simulink model "asservisement_corrige"  (R2019a)
settings: Solver=VariableStepAuto  StartTime=0.0  StopTime=60000000  RelTol=1e-3
model workspace (MAT data in the model file):
  Cx = 0.84
  S = 0.04
libraries: fl_lib x9, nesl_utility x8, sh_lib x5, ee_lib x4, shared3dof x1, simulink x1, dspswit3 x1
settings Model: Creator=Paul  LastModifiedBy=Paul

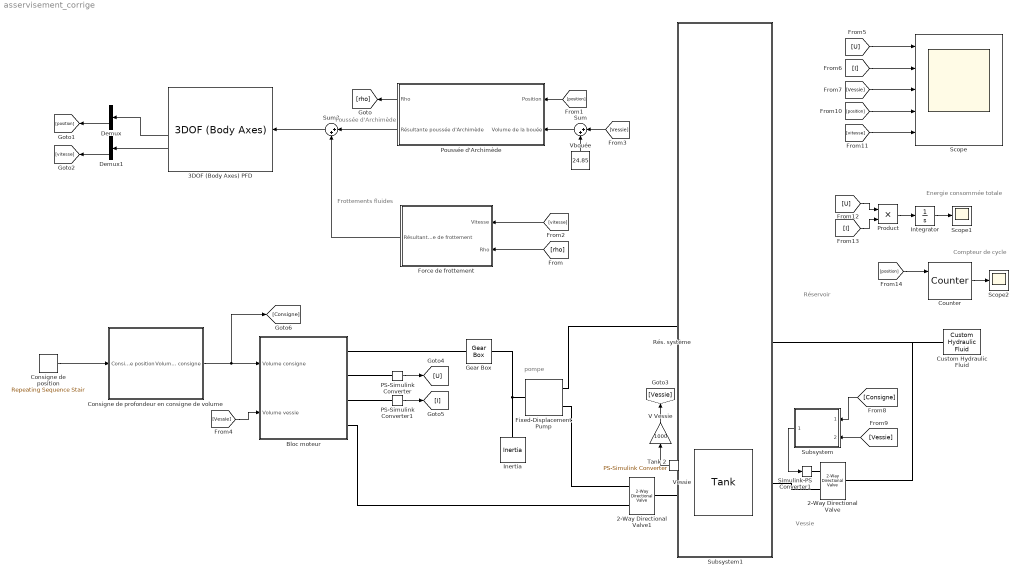
== system asservisement_corrige ==
  note: Vessie
  note: pompe
  note: Energie consommée totale
  note: Compteur de cycle
  note: Poussée d'Archimède
  note: Réservoir
  note: Frottements fluides
  2-Way Directional Valve : sh_lib/Valves/Directional Valves/2-Way Directional Valve  mdl_type=1  area_max=2e-3 m^2  opening_max=0.05 m  opening_tab=[-.002, 0, .002, .005, .015] m  area_tab=[1e-09, 2.0352e-07, 4.0736e-05, .00011438, .00034356] m^2  pressure_tab=[-10000000, -5000000, -2000000, 2000000, 5000000, 10000000] Pa  flow_rate_tab=[-1e-07, -7.0711e-08, -4.4721e-08, 4.4721e-08, 7.0711e-08, 1e-07; -2.0352e-05, -1.4391e-05, -9.1017e-06, 9.1017e-06, 1.4391e-05, 2.0352e-05; -.0040736, -.0028805, -.0018218, .0018218, .0028805, .0040736; -.011438, -.0080879, -.0051152, .0051152, .0080879, .011438; -.034356, -.024293, -.015364, .015364, .024293, .034356] m^3/s  interp_method=1  extrap_method=1  C_d=0.7  x_0=0 m  A_leak=1e-15 m^2  lam_spec=1  B_lam=0.999  Re_cr=12
      settings: SourceProductName=Simscape Fluids  SourceProductBaseCode=SH
  2-Way Directional Valve1 : sh_lib/Valves/Directional Valves/2-Way Directional Valve  mdl_type=1  area_max=2e-2 m^2  opening_max=0.05 m  opening_tab=[-.002, 0, .002, .005, .015] m  area_tab=[1e-09, 2.0352e-07, 4.0736e-05, .00011438, .00034356] m^2  pressure_tab=[-10000000, -5000000, -2000000, 2000000, 5000000, 10000000] Pa  flow_rate_tab=[-1e-07, -7.0711e-08, -4.4721e-08, 4.4721e-08, 7.0711e-08, 1e-07; -2.0352e-05, -1.4391e-05, -9.1017e-06, 9.1017e-06, 1.4391e-05, 2.0352e-05; -.0040736, -.0028805, -.0018218, .0018218, .0028805, .0040736; -.011438, -.0080879, -.0051152, .0051152, .0080879, .011438; -.034356, -.024293, -.015364, .015364, .024293, .034356] m^3/s  interp_method=1  extrap_method=1  C_d=0.7  x_0=0 m  A_leak=1e-15 m^2  lam_spec=1  B_lam=0.999  Re_cr=12
      settings: SourceProductName=Simscape Fluids  SourceProductBaseCode=SH
  "3DOF (Body Axes) PFD " : shared3dof/3DOF (Body Axes)  units=Metric (MKS)  mtype=Fixed  v_ini=0  theta_ini=0  alpha_ini=0  pos_ini=[0 0]  q_ini=0  mass=26  mass_e=0.5  mass_f=3.0  Iyy=1.0  Iyy_e=0.5  Iyy_f=3.0  g_in=Internal  g=9.81  vre_flag=on  abi_flag=off  aMode=0  vel_statename=''  theta_statename=''  pos_statename=''  q_statename=''  mass_statename=''
      settings: SourceProductName=Aerospace Blockset  SourceProductBaseCode=AE
  "Bloc moteur " : Subsystem
  "Consigne de position " : simulink/Sources/Repeating Sequence Stair  OutValues=[0 1000 1000 1000 4000 0].'  tsamp=100000  OutMin=[]  OutMax=[]  OutDataTypeStr=double  OutputDataTypeScalingMode=double  OutDataType=fixdt(0,8)  ConRadixGroup=Best Precision: Vector-wise  OutScaling=2^-12
  Consigne de profondeur en consigne de volume : Subsystem
  Counter : dspswit3/Counter  Direction=Up  CountEvent=Falling edge  CounterSize=User defined  MaxCount=255  InitialCount=0  Output=Count  HitValue=32  ResetInput=on  SamplesPerFrame=1  Ts=1  CntDtype=double  HitDtype=Logical
  Custom Hydraulic Fluid : fl_lib/Hydraulic/Hydraulic Utilities/Custom Hydraulic Fluid  density=850 kg/m^3  viscosity_kin=18e-6 m^2/s  bulk=0.8e9 Pa  alpha=0.005  range_error=2
      settings: SourceProductName=Simscape  SourceProductBaseCode=SS
  Demux : Demux  Outputs=2
  Demux1 : Demux  Outputs=2
  Fixed-Displacement Pump : sh_lib/Pumps and Motors/Fixed-Displacement Pump  D=15 cm^3/rev  loss_spec=1  w_nominal=4 rpm  pr_nominal=400e5 Pa  visc_nominal=18 cSt  dens_nominal=900 kg/m^3  efficiency_vol=0.92  no_load_torque=0.05 N*m  torque_pressure_coeff=0.6e-6 N*m/Pa  p_diff_eff_TLU=[100000, 1000000, 2000000] Pa  omega_eff_TLU=[25, 50, 100, 200, 300, 400] rad/s  vol_eff_TLU=[.816, .908, .954, .977, .981, .984; .325, .663, .831, .916, .925, .946; .137, .568, .78, .892, .893, .91]  mech_eff_TLU=[.996, .996, .996, .996, .996, .996; .988, .989, .989, .989, .989, .99; .981, .981, .982, .982, .983, .984]  p_diff_loss_TLU=[100000, 1000000, 2000000] Pa  omega_loss_TLU=[25, 50, 100, 200, 300, 400] rad/s  vol_loss_TLU=[.023, .023, .023, .023, .0285, .032; .0844, .0842, .0845, .084, .1125, .108; .1079, .108, .11, .108, .1605, .18] * 1e-3 m^3/s  mech_loss_TLU=[.002, .002, .002, .002, .002, .002; .0607, .0556, .0556, .0556, .0556, .0505; .1937, .1937, .1833, .1833, .1729, .1626] N*m  pressure_threshold=1e5 Pa  omega_threshold=10 rad/s  quadrant_check=0  pressure_check=0  min_valid_pressure=0 Pa  vol_eff_min=1e-3  vol_eff_max=1  mech_eff_min=1e-3  mech_eff_max=1
      settings: SourceProductName=Simscape Fluids  SourceProductBaseCode=SH
  Force de frottement : Subsystem
  Gear Box : fl_lib/Mechanical/Mechanisms/Gear Box  ratio=1000  t_in_specify=off  t_in_priority=None  t_in=0 N*m  t_in_nominal_specify=off  t_in_nominal_unit=N*m  t_in_nominal_value=1  t_out_specify=off  t_out_priority=None  t_out=0 N*m  t_out_nominal_specify=off  t_out_nominal_unit=N*m  t_out_nominal_value=1
  Inertia : fl_lib/Mechanical/Rotational Elements/Inertia  inertia=200 g*cm^2  w_specify=off  w_priority=High  w=0 rad/s  w_nominal_specify=off  w_nominal_unit=rad/s  w_nominal_value=1  t_specify=off  t_priority=None  t=0 N*m  t_nominal_specify=off  t_nominal_unit=N*m  t_nominal_value=1
  Integrator : Integrator
  PS-Simulink Converter : nesl_utility/PS-Simulink Converter  PhysicalDomain=network_engine_domain  SubClassName=ps_output  LeftPortType=input  RightPortType=output  PseudoPeriodic=off  Frequencies=[]  Unit=1  AffineConversion=off
  PS-Simulink Converter1 : nesl_utility/PS-Simulink Converter  PhysicalDomain=network_engine_domain  SubClassName=ps_output  LeftPortType=input  RightPortType=output  PseudoPeriodic=off  Frequencies=[]  Unit=1  AffineConversion=off
  Poussée d'Archimède : Subsystem
  Product : Product
  Rés. système : sh_lib/Low-Pressure Blocks/Tank  press=1 bar  level_spec=1  tank_area=0.8 m^2  fluid_volume_tab=[0, .0028, .0065, .0114, .0176, .0252, .0344, .0436, .0512, .0574, .0623, .066, .0688, .0707, .072, .0727] m^3  fluid_level_tab=[0, .02, .04, .06, .08, .1, .12, .14, .16, .18, .2, .22, .24, .26, .28, .3] m  interp_method=1  extrap_method=1  pipe_diam=0.02 m  loss_coeff=1.2  g=9.80665 m/s^2  min_level=1e-3 m  fluid_level_check=0  volume_specify=on  volume_priority=High  volume=0 l  volume_nominal_specify=off  volume_nominal_unit=l  volume_nominal_value=1  level_specify=off  level_priority=None  level=0.025 m  level_nominal_specify=off  level_nominal_unit=m  level_nominal_value=1  pipe_diam_A=0.02 m  loss_coeff_A=1.2  height_B=0.8 m  pipe_diam_B=0.02 m  loss_coeff_B=1.2  height_C=0.8 m  pipe_diam_C=0.02 m  loss_coeff_C=1.2
      settings: SourceProductName=Simscape Fluids  SourceProductBaseCode=SH
  Scope : Scope  NumInputPorts=5
  Scope1 : Scope
  Scope2 : Scope
  Simulink-PS Converter1 : nesl_utility/Simulink-PS Converter  PhysicalDomain=network_engine_domain  SubClassName=ps_input  LeftPortType=input  RightPortType=output  PseudoPeriodic=off  Frequencies=[]  NoiseDistribution=none  NoiseParameters=[]  Unit=m  AffineConversion=off  FilteringAndDerivatives=provide  SimscapeFilterOrder=1  InputFilterTimeConstant=0.001  UdotUserProvided=0
  Subsystem : Subsystem
  Subsystem1 : Subsystem
      mask Display: image('D:\Paul\Documents\TIPE\matlab\Les+flotteurs+Argo2.jpg');
  Sum : Sum  Inputs=|++
  Sum3 : Sum  Inputs=|++
  Tank 2 : nesl_utility/PS-Simulink Converter  PhysicalDomain=network_engine_domain  SubClassName=ps_output  LeftPortType=input  RightPortType=output  PseudoPeriodic=off  Frequencies=[]  Unit=1  AffineConversion=off
  V Vessie : Gain  Gain=1000
  Vbouée : Constant  Value=24.85
  Vessie : sh_lib/Low-Pressure Blocks/Tank  press=400 bar  level_spec=1  tank_area=0.8 m^2  fluid_volume_tab=[0, .0028, .0065, .0114, .0176, .0252, .0344, .0436, .0512, .0574, .0623, .066, .0688, .0707, .072, .0727] m^3  fluid_level_tab=[0, .02, .04, .06, .08, .1, .12, .14, .16, .18, .2, .22, .24, .26, .28, .3] m  interp_method=1  extrap_method=1  pipe_diam=0.02 m  loss_coeff=1.2  g=9.80665 m/s^2  min_level=1e-3 m  fluid_level_check=1  volume_specify=on  volume_priority=High  volume=0.45 l  volume_nominal_specify=off  volume_nominal_unit=l  volume_nominal_value=1  level_specify=off  level_priority=None  level=0.025 m  level_nominal_specify=off  level_nominal_unit=m  level_nominal_value=1  pipe_diam_A=0.02 m  loss_coeff_A=1.2  height_B=0.8 m  pipe_diam_B=0.02 m  loss_coeff_B=1.2  height_C=0.8 m  pipe_diam_C=0.02 m  loss_coeff_C=1.2
      settings: SourceProductName=Simscape Fluids  SourceProductBaseCode=SH
  wires:
  [U] -> Product/1
  Tank 2/1 -> V Vessie/1
  [position] -> Scope/4
  Sum/1 -> Poussée d'Archimède/2(Volume de la bouée)
  Demux/2 -> [position]
  Integrator/1 -> Scope1/1
  Vbouée/1 -> Sum/2
  Force de frottement/1(Résultante force de frottement) -> Sum3/2
  Product/1 -> Integrator/1
  PS-Simulink Converter/1 -> [U]
  [Vessie] -> Subsystem/2(Volume vessie)
  Subsystem/1(Consigne vanne) -> Simulink-PS Converter1/1
  "Consigne de position "/1 -> Consigne de profondeur en consigne de volume/1(Consigne de position)
  [rho] -> Force de frottement/2(Rho)
  "3DOF (Body Axes) PFD "/5 -> Demux1/1
  [I] -> Scope/2
  [I] -> Product/2
  Poussée d'Archimède/2(Résultante poussée d'Archimède) -> Sum3/1
  [position] -> Poussée d'Archimède/1(Position)
  V Vessie/1 -> [Vessie]
  Consigne de profondeur en consigne de volume/1(Volume consigne) -> [Consigne], "Bloc moteur "/1(Volume consigne)
  Poussée d'Archimède/1("Rho ") -> [rho]
  Sum3/1 -> "3DOF (Body Axes) PFD "/2
  [U] -> Scope/1
  [Vessie] -> Sum/1
  [Vessie] -> Scope/3
  "3DOF (Body Axes) PFD "/4 -> Demux/1
  [Vessie] -> "Bloc moteur "/2(Volume vessie)
  [vitesse] -> Scope/5
  [vitesse] -> Force de frottement/1(Vitesse)
  PS-Simulink Converter1/1 -> [I]
  [Consigne] -> Subsystem/1(Volume consigne)
  Demux1/2 -> [vitesse]
  [position] -> Counter/1
  Counter/1 -> Scope2/1
  connections:
  Inertia/LConn1 -- Gear Box/RConn1 -- Fixed-Displacement Pump/LConn1
  Rés. système/LConn1 -- 2-Way Directional Valve/RConn1 -- Custom Hydraulic Fluid/RConn1
  2-Way Directional Valve1/LConn2 -- Fixed-Displacement Pump/RConn1
  Rés. système/RConn2 -- Fixed-Displacement Pump/RConn2
  Simulink-PS Converter1/RConn1 -- 2-Way Directional Valve/LConn1
  Vessie/RConn1 -- Tank 2/LConn1
  Vessie/RConn2 -- 2-Way Directional Valve1/RConn1
  "Bloc moteur "/RConn1 -- Gear Box/LConn1
  Vessie/LConn1 -- 2-Way Directional Valve/LConn2
  2-Way Directional Valve1/LConn1 -- "Bloc moteur "/RConn4
  "Bloc moteur "/RConn2 -- PS-Simulink Converter/LConn1
  PS-Simulink Converter1/LConn1 -- "Bloc moteur "/RConn3

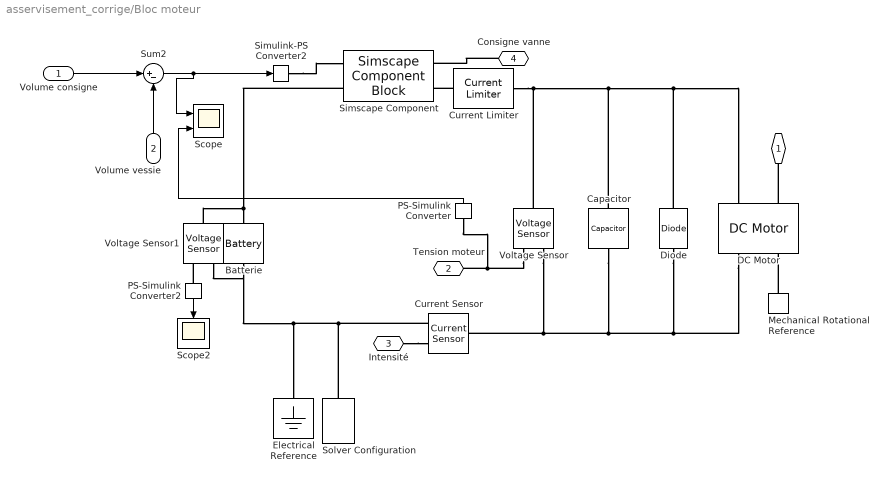
== system asservisement_corrige/Bloc moteur  ==
  Volume consigne : Inport
  Volume vessie : Inport  Port=2
  Batterie : ee_lib/Sources/Battery  Vnom=12 V  R1=0.06 Ohm  prm_AH=2  AH=40 hr*A  V1=10.6 V  AH1=2 hr*A  prm_R2=1  R2=2e+3 Ohm  prm_dyn=1  Rp1=0.005 Ohm  tau1=30 s  Rp2=0.005 Ohm  tau2=30 s  Rp3=0.005 Ohm  tau3=30 s  Rp4=0.005 Ohm  tau4=30 s  Rp5=0.005 Ohm  tau5=30 s  prm_fade=1  N_fade=100  AH_fade=45 hr*A  R1_fade=2.02 Ohm  V1_fade=10.35 V  i_specify=off  i_priority=None  i=0 A  i_nominal_specify=off  i_nominal_unit=A  i_nominal_value=1  v_specify=off  v_priority=None  v=0 V  v_nominal_specify=off  v_nominal_unit=V  v_nominal_value=1  charge_specify=on  charge_priority=High  charge=40 hr*A  charge_nominal_specify=off  charge_nominal_unit=hr*A  charge_nominal_value=1  num_cycles_specify=off  num_cycles_priority=High  num_cycles=0  num_cycles_nominal_specify=off  num_cycles_nominal_unit=1  num_cycles_nominal_value=1  thermal_mass=30000 J/K  Tmeas=298.15 K  Vnom_T2=12 V  R1_T2=2.2 Ohm  V1_T2=11.4 V  R2_T2=2200 Ohm  Rp1_T2=0.005 Ohm  tau1_T2=30 s  Rp2_T2=0.005 Ohm  tau2_T2=30 s  Rp3_T2=0.005 Ohm  tau3_T2=30 s  Rp4_T2=0.005 Ohm  tau4_T2=30 s  Rp5_T2=0.005 Ohm  tau5_T2=30 s  Tmeas2=273.15 K  temperature_specify=off  temperature_priority=High  temperature=298.15 K  temperature_nominal_specify=off  temperature_nominal_unit=K  temperature_nominal_value=1
      settings: SourceProductName=Simscape Electrical
  Capacitor : fl_lib/Electrical/Electrical Elements/Capacitor  c=1000e-6 F  r=1e-6 Ohm  g=0 1/Ohm  i_specify=off  i_priority=None  i=0 A  i_nominal_specify=off  i_nominal_unit=A  i_nominal_value=1  v_specify=off  v_priority=None  v=0 V  v_nominal_specify=off  v_nominal_unit=V  v_nominal_value=1  vc_specify=off  vc_priority=High  vc=0 V  vc_nominal_specify=off  vc_nominal_unit=V  vc_nominal_value=1
  Current Limiter : ee_lib/Semiconductors & Converters/Current Limiter  iLim=50 A  vLim=0.1 V  gLim=1e-3 1/Ohm  thermal_mass=100 J/K  initial_temperature=298.15 K
      settings: SourceProductName=Simscape Electrical  SourceProductBaseCode=PS
  Current Sensor : fl_lib/Electrical/Electrical Sensors/Current Sensor
  DC Motor : ee_lib/Electromechanical/Brushed Motors/DC Motor  parameterization=3  Ra=10 Ohm  La=0.0001 H  emf_or_torque=1  Kv=0.1 V/rpm  Ki=6.876e-4 N*m/A  T_stall=0.24e-3 N*m  w_max=5000 rpm  w_rated=4000 rpm  P_rated=400 W  V_rated=12 V  J=2000 g*cm^2  lam_param=1  lam=1e-6 N*m/(rad/s)  i_noload=0 A  V_i_noload=1.5 V  speed0=0 rpm  alpha=3.93e-3 1/K  Tmeas=25 degC  thermal_mass=100 J/K  initial_temperature=25 degC
      settings: SourceProductName=Simscape Electrical
  Diode : ee_lib/Semiconductors & Converters/Diode  ModelType=ee.enum.diode.modelType.pwl  Vf=0.1 V  Ron=0.3 Ohm  Goff=1e-8 S  prmExp=ee.enum.diode.expParam.useTwo  I12=[.0137, .545] A  V12=[.6, .7] V  IS=1e-12 A  ec=1  I1=0.0137 A  V1=0.6 V  RS=0 Ohm  Tmeas=25 degC  N_series=1  N_parallel=1  Rz=0.3 Ohm  BV=inf V  C_param=ee.enum.diode.capParam.fixed  CJ=5 pF  CJ0=5 pF  VJ=1 V  Mgrad=0.5  Vvec=[.1, 10, 100] V  Cvec=[3.5, 1, .4] pF  FC=0.5  Q_param=ee.enum.diode.recoveryParam.off  iRM=-7.15 A  iF=4 A  didt=-750 A/us  trr_factor=3  trr=115 ns  Qrr=1500 s*uA  TT=50 ns  tau=100 ns  T_param=ee.enum.diode.temperatureParam.off  IS_T2=1.25e-7 A  I1_T2=0.245 A  V1_T2=0.5 V  Tmeas2=125 degC  EG_param=ee.enum.diode.egapParam.material_si  EG=1.11 eV  XTI_param=ee.enum.diode.xtiParam.pn  XTI=3  dBVdT=0 V/K  Tdevice=25 degC  i_specify=off  i_priority=None  i=0 A  i_nominal_specify=off  i_nominal_unit=A  i_nominal_value=1  v_specify=off  v_priority=None  v=0 V  v_nominal_specify=off  v_nominal_unit=V  v_nominal_value=1  i_capacitor_specify=off  i_capacitor_priority=None  i_capacitor=0 A  i_capacitor_nominal_specify=off  i_capacitor_nominal_unit=A  i_capacitor_nominal_value=1  v_capacitor_specify=off  v_capacitor_priority=None  v_capacitor=0 V  v_capacitor_nominal_specify=off  v_capacitor_nominal_unit=V  v_capacitor_nominal_value=1  power_dissipated_specify=off  power_dissipated_priority=None  power_dissipated=0 W  power_dissipated_nominal_specify=off  power_dissipated_nominal_unit=W  power_dissipated_nominal_value=1  Rth=[0, 10] K/W  thermal_mass_parameterization=ee.enum.thermalNetwork.timeconstant  thermal_mass=[0, 1] J/K  thermal_time_constant=[0, 10] s  thermal_mass_initial_temperatures=[25, 25] degC
      settings: SourceProductName=Simscape Electrical
  Electrical Reference : fl_lib/Electrical/Electrical Elements/Electrical Reference
  Mechanical Rotational Reference : fl_lib/Mechanical/Rotational Elements/Mechanical Rotational Reference
  PS-Simulink Converter : nesl_utility/PS-Simulink Converter  PhysicalDomain=network_engine_domain  SubClassName=ps_output  LeftPortType=input  RightPortType=output  PseudoPeriodic=off  Frequencies=[]  Unit=1  AffineConversion=off
  PS-Simulink Converter2 : nesl_utility/PS-Simulink Converter  PhysicalDomain=network_engine_domain  SubClassName=ps_output  LeftPortType=input  RightPortType=output  PseudoPeriodic=off  Frequencies=[]  Unit=1  AffineConversion=off
  Scope : Scope  NumInputPorts=2
  Scope2 : Scope
  Simscape Component : SimscapeComponentBlock  SourceFile=delayed_switch  ComponentPath=delayed_switch  ComponentVariants=delayed_switch  ComponentVariantNames=delayed_switch  ClassName=delayed_switch  SchemaVersion=1  R_closed=0.01 Ohm  G_open=1e-8 1/Ohm  T_closed=0.001  T_open=-0.001  InitMode=switching.open  i_specify=off  i_priority=None  i=0 A  i_nominal_specify=off  i_nominal_unit=A  i_nominal_value=1  v_specify=off  v_priority=None  v=0 V  v_nominal_specify=off  v_nominal_unit=V  v_nominal_value=1
      settings: CopyFcn=simscape.engine.sli.internal.componentblockcallback(gcbh,'COPY')  PreCopyFcn=simscape.engine.sli.internal.componentblockcallback(gcbh,'PRECOPY')  PreDeleteFcn=simscape.engine.sli.internal.componentblockcallback(gcbh,'PREDELETE')
      mask Type: Switch with Hysteresis
  Simulink-PS Converter2 : nesl_utility/Simulink-PS Converter  PhysicalDomain=network_engine_domain  SubClassName=ps_input  LeftPortType=input  RightPortType=output  PseudoPeriodic=off  Frequencies=[]  NoiseDistribution=none  NoiseParameters=[]  Unit=V  AffineConversion=off  FilteringAndDerivatives=provide  SimscapeFilterOrder=1  InputFilterTimeConstant=0.001  UdotUserProvided=0
  Solver Configuration : nesl_utility/Solver Configuration  PhysicalDomain=network_engine_domain  SubClassName=solver  LeftPortType=input  RightPortType=generic  Tones=[]  Harmonics=[]  SimulateNoise=off  Profile=off  UseLocalSampling=off  EnableSwitchedLinearOptims=on  FrequencyDomain=off  UseCCode=off  RelTol=0.001  AbsTol=1e-06  MinStep=1e-09  ToWorkspace=off  RevertToSquareIcSolve=off  NumHomotopyIterations=100  PhasorMode=off  PhasorModeNumHarmonics=1  DoDC=off  ResidualTolerance=1e-09  UseLocalSolver=off  LocalSolverChoice=NE_BACKWARD_EULER_ADVANCER  LocalSolverSampleTime=0.001  DoFixedCost=off  MaxNonlinIter=3  MaxModeIter=2  LinearAlgebra=auto  EquationFormulation=NE_TIME_EF  DelaysMemoryBudget=1024  AutomaticFiltering=on  FilteringTimeConstant=0.001  PartitionStorageMethod=AS_NEEDED  PartitionMemoryBudget=1024  PartitionMethod=ROBUST
  Sum2 : Sum  Inputs=|+-
  Voltage Sensor : fl_lib/Electrical/Electrical Sensors/Voltage Sensor
  Voltage Sensor1 : fl_lib/Electrical/Electrical Sensors/Voltage Sensor
  " " : PMIOPort  Side=Right
  Tension moteur : PMIOPort  Port=2  Side=Right
  Intensité : PMIOPort  Port=3  Side=Right
  Consigne vanne : PMIOPort  Port=4  Side=Right
  wires:
  PS-Simulink Converter2/1 -> Scope2/1
  Sum2/1 -> Scope/1, Simulink-PS Converter2/1
  Volume vessie/1 -> Sum2/2
  Volume consigne/1 -> Sum2/1
  PS-Simulink Converter/1 -> Scope/2
  connections:
  PS-Simulink Converter2/LConn1 -- Voltage Sensor1/RConn1
  Solver Configuration/RConn1 -- Current Sensor/RConn2 -- Voltage Sensor1/RConn2 -- Batterie/RConn1 -- Electrical Reference/LConn1
  DC Motor/LConn2 -- " "/RConn1
  Simulink-PS Converter2/RConn1 -- Simscape Component/LConn1
  Batterie/LConn1 -- Simscape Component/LConn2 -- Voltage Sensor1/LConn1
  Current Limiter/LConn1 -- Simscape Component/RConn2
  Intensité/RConn1 -- Current Sensor/RConn1
  Mechanical Rotational Reference/LConn1 -- DC Motor/RConn2
  Voltage Sensor/RConn1 -- PS-Simulink Converter/LConn1 -- Tension moteur/RConn1
  Current Limiter/RConn1 -- Voltage Sensor/LConn1 -- Capacitor/LConn1 -- Diode/RConn1 -- DC Motor/LConn1
  DC Motor/RConn1 -- Diode/LConn1 -- Capacitor/RConn1 -- Voltage Sensor/RConn2 -- Current Sensor/LConn1
  Consigne vanne/RConn1 -- Simscape Component/RConn1

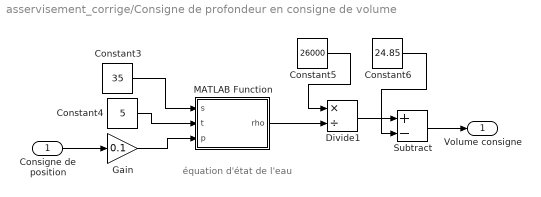
== system asservisement_corrige/Consigne de profondeur en consigne de volume ==
  note: équation d'état de l'eau
  Consigne de position : Inport
  Constant3 : Constant  Value=35
  Constant4 : Constant  Value=5
  Constant5 : Constant  Value=26000
  Constant6 : Constant  Value=24.85
  Divide1 : Product  Inputs=*/
  Gain : Gain  Gain=0.1
  MATLAB Function : MATLAB Function  TreatAsAtomicUnit=on
  Subtract : Sum  Inputs=+-
  Volume consigne : Outport
  wires:
  Constant4/1 -> MATLAB Function/2(t)
  Divide1/1 -> Subtract/1
  Gain/1 -> MATLAB Function/3(p)
  Subtract/1 -> Volume consigne/1
  Constant5/1 -> Divide1/1
  MATLAB Function/1(rho) -> Divide1/2
  Constant6/1 -> Subtract/2
  Constant3/1 -> MATLAB Function/1(s)
  Consigne de position/1 -> Gain/1

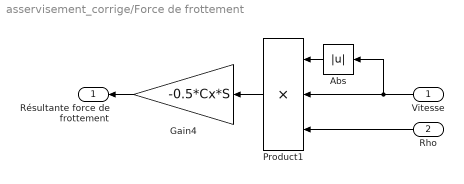
== system asservisement_corrige/Force de frottement ==
  Vitesse : Inport
  Rho : Inport  Port=2
  Abs : Abs
  Gain4 : Gain  Gain=-0.5*Cx*S
  Product1 : Product  Inputs=3
  Résultante force de frottement : Outport
  wires:
  Product1/1 -> Gain4/1
  Abs/1 -> Product1/1
  Gain4/1 -> Résultante force de frottement/1
  Rho/1 -> Product1/3
  Vitesse/1 -> Abs/1, Product1/2

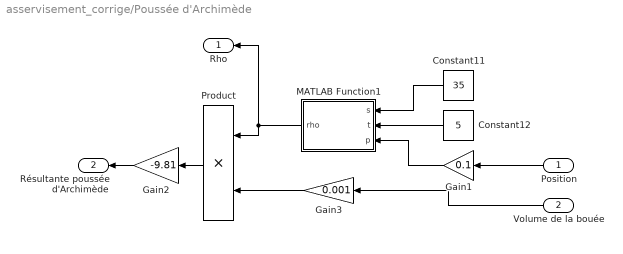
== system asservisement_corrige/Poussée d'Archimède ==
  Position : Inport
  Volume de la bouée : Inport  Port=2
  Constant11 : Constant  Value=35
  Constant12 : Constant  Value=5
  Gain1 : Gain  Gain=0.1
  Gain2 : Gain  Gain=-9.81
  Gain3 : Gain  Gain=0.001
  MATLAB Function1 : MATLAB Function  TreatAsAtomicUnit=on
  Product : Product
  "Rho " : Outport
  Résultante poussée d'Archimède : Outport  Port=2
  wires:
  Position/1 -> Gain1/1
  Constant11/1 -> MATLAB Function1/1(s)
  MATLAB Function1/1(rho) -> "Rho "/1, Product/1
  Gain1/1 -> MATLAB Function1/3(p)
  Product/1 -> Gain2/1
  Constant12/1 -> MATLAB Function1/2(t)
  Gain3/1 -> Product/2
  Volume de la bouée/1 -> Gain3/1
  Gain2/1 -> Résultante poussée d'Archimède/1

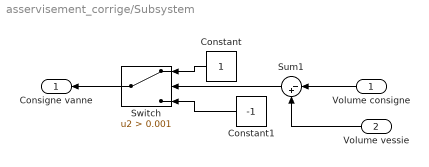
== system asservisement_corrige/Subsystem ==
  Volume consigne : Inport
  Volume vessie : Inport  Port=2
  Constant : Constant
  Constant1 : Constant  Value=-1
  Sum1 : Sum  Inputs=|-+
  Switch : Switch  Criteria=u2 > Threshold  Threshold=0.001
  Consigne vanne : Outport
  wires:
  Constant/1 -> Switch/1
  Volume consigne/1 -> Sum1/1
  Sum1/1 -> Switch/2
  Constant1/1 -> Switch/3
  Volume vessie/1 -> Sum1/2
  Switch/1 -> Consigne vanne/1

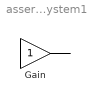
== system asservisement_corrige/Subsystem1 ==
  Gain : Gain
  wires:
  ? -> Gain/1
  Gain/1 -> ?

== matlab function asservisement_corrige/Poussée d'Archimède/MATLAB Function1 ==
  data: s input; rho output; t input; p input
function rho=ies80(s,t,p)

% 
% International Equation of State of sea water : rho=ies80(s,t,p)
%   rho  density     (kg/m3)
%    s   salinity
%    t   temperature (°C)
%    p   pressure    (bars)
%
%    rho,s,t,p can be vector or matrix
%
%    rho=ies80(s,t) use p=0
%
%-----------------------------------
% Olivier Le Calvé 
% E-mail : lecalve@isitv.univ-tln.fr
%-----------------------------------

r0_coef=[999.842594,6.793952e-2,-9.09529e-3,1.001685e-4,-1.120083e-6,...
         6.536332e-9,8.24493e-1,-4.0899e-3,7.6438e-5,-8.2467e-7,...
         5.3875e-9,-5.72466e-3,1.0227e-4,-1.6546e-6,4.8314e-4];

r0=polyval(r0_coef(6:-1:1),t)+...
   polyval(r0_coef(11:-1:7),t).*s+...
   polyval(r0_coef(14:-1:12),t).*s.^1.5+...
   r0_coef(15)*s.^2;

if nargin==3

K_coef=[19652.21,148.4206,-2.327105,1.360447e-2,-5.155288e-5,3.239908,...
        1.43713e-3,1.16092e-4,-5.77905e-7,8.50935e-5,...
        -6.12293e-6,5.2787e-8,54.6746,-0.603459,1.09987e-2,...
        -6.1670e-5,7.944e-2,1.6483e-2,-5.3009e-4,2.2838e-3,...
        -1.0981e-5,-1.6078e-6,1.91075e-4,-9.9348e-7,...
        2.0816e-8,9.1697e-10];

K=polyval(K_coef(5:-1:1),t)+...
  polyval(K_coef(9:-1:6),t).*p+...
  polyval(K_coef(12:-1:10),t).*p.^2+...
  polyval(K_coef(16:-1:13),t).*s+...
  polyval(K_coef(19:-1:17),t).*s.^1.5+...
  polyval(K_coef(22:-1:20),t).*p.*s+...
  K_coef(23)*p.*s.^1.5+...
  polyval(K_coef(26:-1:24),t).*p.^2.*s;
  
rho=r0./(1-p./K);

else

rho=r0;

end

== matlab function asservisement_corrige/Consigne de profondeur en consigne de volume/MATLAB Function ==
  data: s input; rho output; t input; p input
function rho=ies80(s,t,p)

% 
% International Equation of State of sea water : rho=ies80(s,t,p)
%   rho  density     (kg/m3)
%    s   salinity
%    t   temperature (°C)
%    p   pressure    (bars)
%
%    rho,s,t,p can be vector or matrix
%
%    rho=ies80(s,t) use p=0
%
%-----------------------------------
% Olivier Le Calvé 
% E-mail : lecalve@isitv.univ-tln.fr
%-----------------------------------

r0_coef=[999.842594,6.793952e-2,-9.09529e-3,1.001685e-4,-1.120083e-6,...
         6.536332e-9,8.24493e-1,-4.0899e-3,7.6438e-5,-8.2467e-7,...
         5.3875e-9,-5.72466e-3,1.0227e-4,-1.6546e-6,4.8314e-4];

r0=polyval(r0_coef(6:-1:1),t)+...
   polyval(r0_coef(11:-1:7),t).*s+...
   polyval(r0_coef(14:-1:12),t).*s.^1.5+...
   r0_coef(15)*s.^2;

if nargin==3

K_coef=[19652.21,148.4206,-2.327105,1.360447e-2,-5.155288e-5,3.239908,...
        1.43713e-3,1.16092e-4,-5.77905e-7,8.50935e-5,...
        -6.12293e-6,5.2787e-8,54.6746,-0.603459,1.09987e-2,...
        -6.1670e-5,7.944e-2,1.6483e-2,-5.3009e-4,2.2838e-3,...
        -1.0981e-5,-1.6078e-6,1.91075e-4,-9.9348e-7,...
        2.0816e-8,9.1697e-10];

K=polyval(K_coef(5:-1:1),t)+...
  polyval(K_coef(9:-1:6),t).*p+...
  polyval(K_coef(12:-1:10),t).*p.^2+...
  polyval(K_coef(16:-1:13),t).*s+...
  polyval(K_coef(19:-1:17),t).*s.^1.5+...
  polyval(K_coef(22:-1:20),t).*p.*s+...
  K_coef(23)*p.*s.^1.5+...
  polyval(K_coef(26:-1:24),t).*p.^2.*s;
  
rho=r0./(1-p./K);

else

rho=r0;

end
